simulink model "crane_sm"  (R2026a)
settings: Solver=ode23t  StopTime=8
undefined symbols (not defined in the file): ctrl_centerDamping, ctrl_centerGain, ctrl_clearanceMargin, ctrl_forceMax, ctrl_K, ctrl_lqrScale, ctrl_pendulumLength, ctrl_postClearDamping, ctrl_postClearGain, ctrl_pumpControlAmplitude, ctrl_pumpControlDuration, ctrl_pumpControlPhase, ctrl_pumpFrequency, ctrl_targetX, ctrl_transferClearance, ctrl_transferDamping, ctrl_transferForce, ctrl_wallTop, ctrl_wallX, X, Y, Z
libraries: sm_lib x18, nesl_utility x10
settings Model: DataDictionary=craneDD.sldd  Creator=grouleau  LastModifiedBy=grouleau

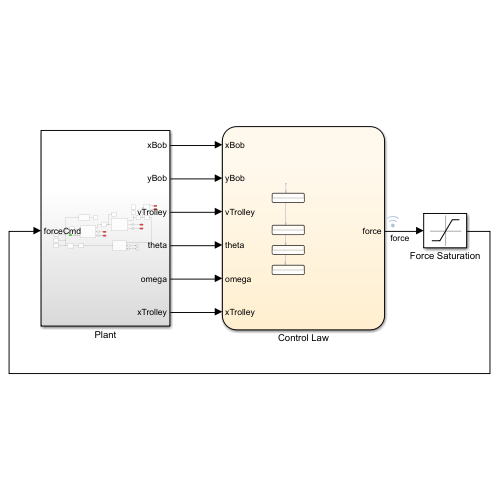
[thumbnail: Simulink's stored preview of the top-level diagram]
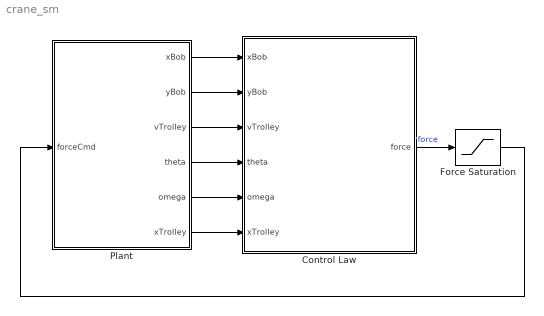
== system crane_sm ==
  Control Law : Stateflow chart  TreatAsAtomicUnit=on
  Force Saturation : Saturate  UpperLimit=60  LowerLimit=-60
  Plant : Subsystem
  wires:
  Plant/6(xTrolley) -> Control Law/6(xTrolley)
  Plant/5(omega) -> Control Law/5(omega)
  Control Law/1(force) -> Force Saturation/1  "force"
  Plant/4(theta) -> Control Law/4(theta)
  Plant/2(yBob) -> Control Law/2(yBob)
  Plant/3(vTrolley) -> Control Law/3(vTrolley)
  Plant/1(xBob) -> Control Law/1(xBob)
  Force Saturation/1 -> Plant/1(forceCmd)

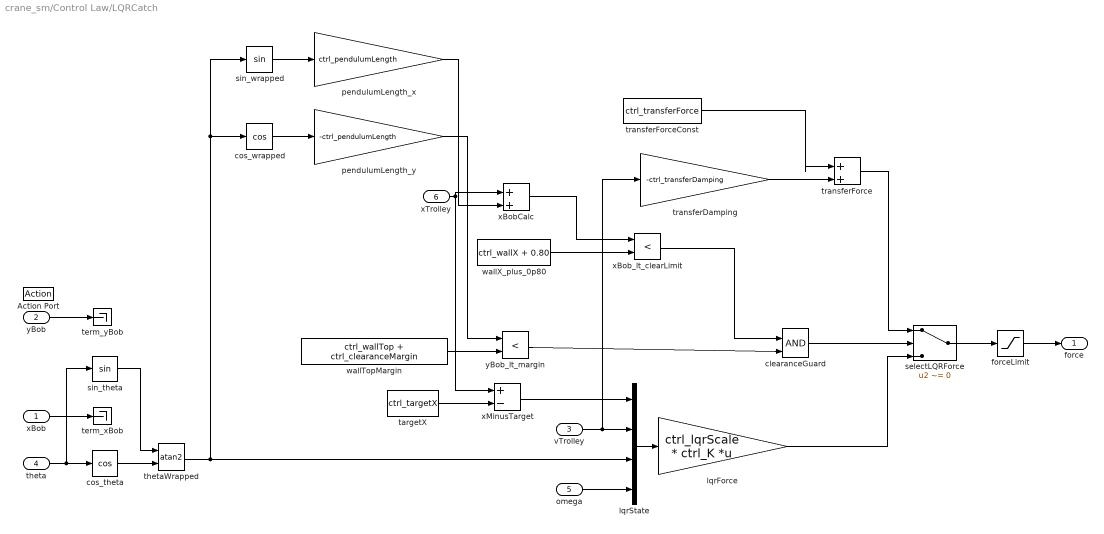
== system crane_sm/Control Law/LQRCatch ==
  xBob : Inport
  yBob : Inport  Port=2
  vTrolley : Inport  Port=3
  theta : Inport  Port=4
  omega : Inport  Port=5
  xTrolley : Inport  Port=6
  Action Port : ActionPort
      settings: CopyFcn=Stateflow.SLINSF.SimulinkMan.removeBlockPreDeleteFcn  PreDeleteFcn=Stateflow.SLINSF.SimulinkMan.unsafePredeleteFcn
  clearanceGuard : Logic  IconShape=distinctive  AllPortsSameDT=off  OutDataTypeStr=boolean
  cos_theta : Trigonometry  Operator=cos
  cos_wrapped : Trigonometry  Operator=cos
  forceLimit : Saturate  UpperLimit=ctrl_forceMax  LowerLimit=-ctrl_forceMax
  lqrForce : Gain  Gain=ctrl_lqrScale * ctrl_K  Multiplication=Matrix(K*u)
  lqrState : Mux
  pendulumLength_x : Gain  Gain=ctrl_pendulumLength
  pendulumLength_y : Gain  Gain=-ctrl_pendulumLength
  selectLQRForce : Switch  Criteria=u2 ~= 0  SaturateOnIntegerOverflow=off  InputSameDT=off
  sin_theta : Trigonometry
  sin_wrapped : Trigonometry
  targetX : Constant  Value=ctrl_targetX
  term_xBob : Terminator
  term_yBob : Terminator
  thetaWrapped : Trigonometry  Operator=atan2
  transferDamping : Gain  Gain=-ctrl_transferDamping
  transferForce : Sum  Inputs=|++
  transferForceConst : Constant  Value=ctrl_transferForce
  wallTopMargin : Constant  Value=ctrl_wallTop + ctrl_clearanceMargin
  wallX_plus_0p80 : Constant  Value=ctrl_wallX + 0.80
  xBobCalc : Sum  Inputs=|++
  xBob_lt_clearLimit : RelationalOperator  Operator=<  OutDataTypeStr=boolean  RndMeth=Simplest  InputSameDT=off
  xMinusTarget : Sum  Inputs=+-
  yBob_lt_margin : RelationalOperator  Operator=<  OutDataTypeStr=boolean  RndMeth=Simplest  InputSameDT=off
  force : Outport
  wires:
  yBob/1 -> term_yBob/1
  xBob/1 -> term_xBob/1
  omega/1 -> lqrState/4
  theta/1 -> sin_theta/1, cos_theta/1
  sin_theta/1 -> thetaWrapped/1
  thetaWrapped/1 -> sin_wrapped/1, cos_wrapped/1, lqrState/3
  sin_wrapped/1 -> pendulumLength_x/1
  cos_theta/1 -> thetaWrapped/2
  cos_wrapped/1 -> pendulumLength_y/1
  pendulumLength_x/1 -> xBobCalc/2
  wallX_plus_0p80/1 -> xBob_lt_clearLimit/2
  pendulumLength_y/1 -> yBob_lt_margin/1
  forceLimit/1 -> force/1
  xTrolley/1 -> xBobCalc/1, xMinusTarget/1
  xBob_lt_clearLimit/1 -> clearanceGuard/1
  wallTopMargin/1 -> yBob_lt_margin/2
  transferForce/1 -> selectLQRForce/1
  transferDamping/1 -> transferForce/2
  targetX/1 -> xMinusTarget/2
  xBobCalc/1 -> xBob_lt_clearLimit/1
  vTrolley/1 -> transferDamping/1, lqrState/2
  clearanceGuard/1 -> selectLQRForce/2
  transferForceConst/1 -> transferForce/1
  yBob_lt_margin/1 -> clearanceGuard/2
  lqrState/1 -> lqrForce/1
  xMinusTarget/1 -> lqrState/1
  lqrForce/1 -> selectLQRForce/3
  selectLQRForce/1 -> forceLimit/1

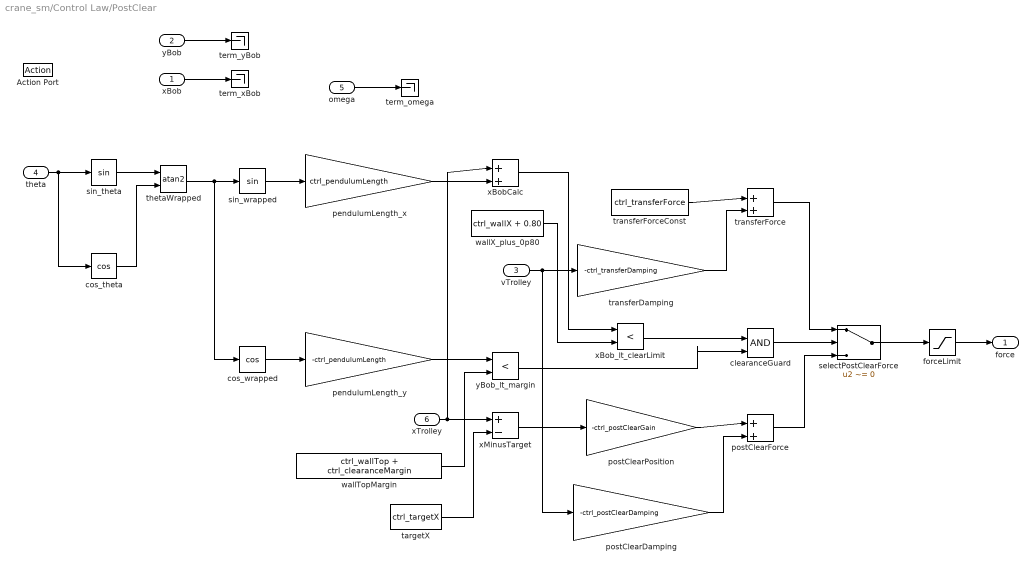
== system crane_sm/Control Law/PostClear ==
  xBob : Inport
  yBob : Inport  Port=2
  vTrolley : Inport  Port=3
  theta : Inport  Port=4
  omega : Inport  Port=5
  xTrolley : Inport  Port=6
  Action Port : ActionPort
      settings: CopyFcn=Stateflow.SLINSF.SimulinkMan.removeBlockPreDeleteFcn  PreDeleteFcn=Stateflow.SLINSF.SimulinkMan.unsafePredeleteFcn
  clearanceGuard : Logic  IconShape=distinctive  AllPortsSameDT=off  OutDataTypeStr=boolean
  cos_theta : Trigonometry  Operator=cos
  cos_wrapped : Trigonometry  Operator=cos
  forceLimit : Saturate  UpperLimit=ctrl_forceMax  LowerLimit=-ctrl_forceMax
  pendulumLength_x : Gain  Gain=ctrl_pendulumLength
  pendulumLength_y : Gain  Gain=-ctrl_pendulumLength
  postClearDamping : Gain  Gain=-ctrl_postClearDamping
  postClearForce : Sum  Inputs=|++
  postClearPosition : Gain  Gain=-ctrl_postClearGain
  selectPostClearForce : Switch  Criteria=u2 ~= 0  SaturateOnIntegerOverflow=off  InputSameDT=off
  sin_theta : Trigonometry
  sin_wrapped : Trigonometry
  targetX : Constant  Value=ctrl_targetX
  term_omega : Terminator
  term_xBob : Terminator
  term_yBob : Terminator
  thetaWrapped : Trigonometry  Operator=atan2
  transferDamping : Gain  Gain=-ctrl_transferDamping
  transferForce : Sum  Inputs=|++
  transferForceConst : Constant  Value=ctrl_transferForce
  wallTopMargin : Constant  Value=ctrl_wallTop + ctrl_clearanceMargin
  wallX_plus_0p80 : Constant  Value=ctrl_wallX + 0.80
  xBobCalc : Sum  Inputs=|++
  xBob_lt_clearLimit : RelationalOperator  Operator=<  OutDataTypeStr=boolean  RndMeth=Simplest  InputSameDT=off
  xMinusTarget : Sum  Inputs=+-
  yBob_lt_margin : RelationalOperator  Operator=<  OutDataTypeStr=boolean  RndMeth=Simplest  InputSameDT=off
  force : Outport
  wires:
  yBob/1 -> term_yBob/1
  xBob/1 -> term_xBob/1
  thetaWrapped/1 -> cos_wrapped/1, sin_wrapped/1
  cos_theta/1 -> thetaWrapped/2
  theta/1 -> sin_theta/1, cos_theta/1
  omega/1 -> term_omega/1
  sin_theta/1 -> thetaWrapped/1
  pendulumLength_x/1 -> xBobCalc/2
  sin_wrapped/1 -> pendulumLength_x/1
  cos_wrapped/1 -> pendulumLength_y/1
  pendulumLength_y/1 -> yBob_lt_margin/1
  xTrolley/1 -> xBobCalc/1, xMinusTarget/1
  xBob_lt_clearLimit/1 -> clearanceGuard/1
  wallX_plus_0p80/1 -> xBob_lt_clearLimit/2
  wallTopMargin/1 -> yBob_lt_margin/2
  xMinusTarget/1 -> postClearPosition/1
  targetX/1 -> xMinusTarget/2
  xBobCalc/1 -> xBob_lt_clearLimit/1
  vTrolley/1 -> transferDamping/1, postClearDamping/1
  clearanceGuard/1 -> selectPostClearForce/2
  yBob_lt_margin/1 -> clearanceGuard/2
  transferForceConst/1 -> transferForce/1
  transferForce/1 -> selectPostClearForce/1
  transferDamping/1 -> transferForce/2
  postClearPosition/1 -> postClearForce/1
  postClearForce/1 -> selectPostClearForce/3
  postClearDamping/1 -> postClearForce/2
  selectPostClearForce/1 -> forceLimit/1
  forceLimit/1 -> force/1

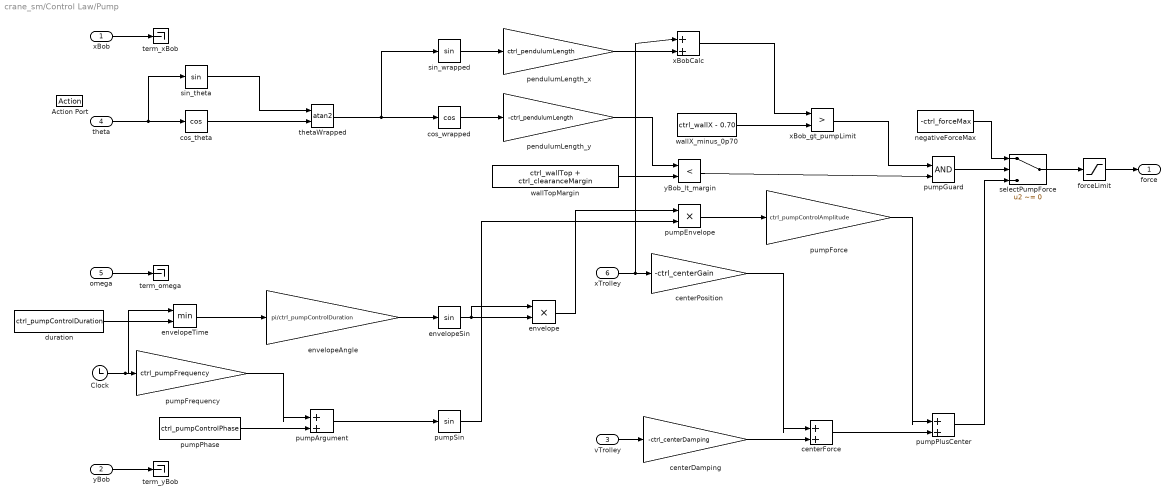
== system crane_sm/Control Law/Pump ==
  xBob : Inport
  yBob : Inport  Port=2
  vTrolley : Inport  Port=3
  theta : Inport  Port=4
  omega : Inport  Port=5
  xTrolley : Inport  Port=6
  Action Port : ActionPort
      settings: CopyFcn=Stateflow.SLINSF.SimulinkMan.removeBlockPreDeleteFcn  PreDeleteFcn=Stateflow.SLINSF.SimulinkMan.unsafePredeleteFcn
  Clock : Clock
  centerDamping : Gain  Gain=-ctrl_centerDamping
  centerForce : Sum  Inputs=|++
  centerPosition : Gain  Gain=-ctrl_centerGain
  cos_theta : Trigonometry  Operator=cos
  cos_wrapped : Trigonometry  Operator=cos
  duration : Constant  Value=ctrl_pumpControlDuration
  envelope : Product
  envelopeAngle : Gain  Gain=pi/ctrl_pumpControlDuration
  envelopeSin : Trigonometry
  envelopeTime : MinMax  Inputs=2
  forceLimit : Saturate  UpperLimit=ctrl_forceMax  LowerLimit=-ctrl_forceMax
  negativeForceMax : Constant  Value=-ctrl_forceMax
  pendulumLength_x : Gain  Gain=ctrl_pendulumLength
  pendulumLength_y : Gain  Gain=-ctrl_pendulumLength
  pumpArgument : Sum  Inputs=|++
  pumpEnvelope : Product
  pumpForce : Gain  Gain=ctrl_pumpControlAmplitude
  pumpFrequency : Gain  Gain=ctrl_pumpFrequency
  pumpGuard : Logic  IconShape=distinctive  AllPortsSameDT=off  OutDataTypeStr=boolean
  pumpPhase : Constant  Value=ctrl_pumpControlPhase
  pumpPlusCenter : Sum  Inputs=|++
  pumpSin : Trigonometry
  selectPumpForce : Switch  Criteria=u2 ~= 0  SaturateOnIntegerOverflow=off  InputSameDT=off
  sin_theta : Trigonometry
  sin_wrapped : Trigonometry
  term_omega : Terminator
  term_xBob : Terminator
  term_yBob : Terminator
  thetaWrapped : Trigonometry  Operator=atan2
  wallTopMargin : Constant  Value=ctrl_wallTop + ctrl_clearanceMargin
  wallX_minus_0p70 : Constant  Value=ctrl_wallX - 0.70
  xBobCalc : Sum  Inputs=|++
  xBob_gt_pumpLimit : RelationalOperator  Operator=>  OutDataTypeStr=boolean  RndMeth=Simplest  InputSameDT=off
  yBob_lt_margin : RelationalOperator  Operator=<  OutDataTypeStr=boolean  RndMeth=Simplest  InputSameDT=off
  force : Outport
  wires:
  duration/1 -> envelopeTime/2
  xBob/1 -> term_xBob/1
  yBob/1 -> term_yBob/1
  pendulumLength_x/1 -> xBobCalc/2
  theta/1 -> sin_theta/1, cos_theta/1
  omega/1 -> term_omega/1
  selectPumpForce/1 -> forceLimit/1
  Clock/1 -> envelopeTime/1, pumpFrequency/1
  sin_theta/1 -> thetaWrapped/1
  cos_theta/1 -> thetaWrapped/2
  envelopeTime/1 -> envelopeAngle/1
  pumpFrequency/1 -> pumpArgument/1
  pumpPhase/1 -> pumpArgument/2
  thetaWrapped/1 -> sin_wrapped/1, cos_wrapped/1
  envelopeSin/1 -> envelope/1, envelope/2
  envelopeAngle/1 -> envelopeSin/1
  pumpSin/1 -> pumpEnvelope/2
  pumpArgument/1 -> pumpSin/1
  sin_wrapped/1 -> pendulumLength_x/1
  cos_wrapped/1 -> pendulumLength_y/1
  xBobCalc/1 -> xBob_gt_pumpLimit/1
  pendulumLength_y/1 -> yBob_lt_margin/1
  wallTopMargin/1 -> yBob_lt_margin/2
  xTrolley/1 -> xBobCalc/1, centerPosition/1
  envelope/1 -> pumpEnvelope/1
  vTrolley/1 -> centerDamping/1
  pumpPlusCenter/1 -> selectPumpForce/3
  wallX_minus_0p70/1 -> xBob_gt_pumpLimit/2
  yBob_lt_margin/1 -> pumpGuard/2
  pumpEnvelope/1 -> pumpForce/1
  centerPosition/1 -> centerForce/1
  centerDamping/1 -> centerForce/2
  xBob_gt_pumpLimit/1 -> pumpGuard/1
  pumpForce/1 -> pumpPlusCenter/1
  centerForce/1 -> pumpPlusCenter/2
  pumpGuard/1 -> selectPumpForce/2
  negativeForceMax/1 -> selectPumpForce/1
  forceLimit/1 -> force/1

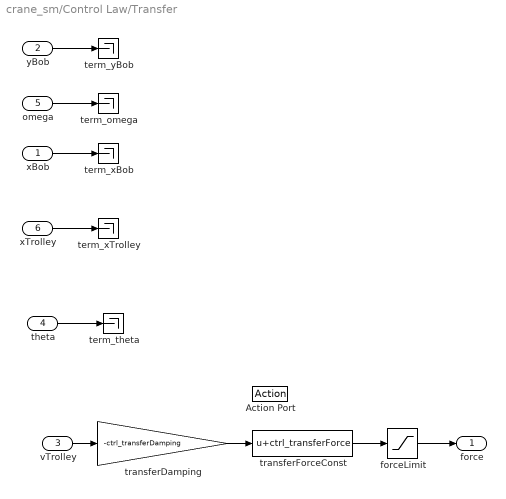
== system crane_sm/Control Law/Transfer ==
  xBob : Inport
  yBob : Inport  Port=2
  vTrolley : Inport  Port=3
  theta : Inport  Port=4
  omega : Inport  Port=5
  xTrolley : Inport  Port=6
  Action Port : ActionPort
      settings: CopyFcn=Stateflow.SLINSF.SimulinkMan.removeBlockPreDeleteFcn  PreDeleteFcn=Stateflow.SLINSF.SimulinkMan.unsafePredeleteFcn
  forceLimit : Saturate  UpperLimit=ctrl_forceMax  LowerLimit=-ctrl_forceMax
  term_omega : Terminator
  term_theta : Terminator
  term_xBob : Terminator
  term_xTrolley : Terminator
  term_yBob : Terminator
  transferDamping : Gain  Gain=-ctrl_transferDamping
  transferForceConst : Bias  Bias=ctrl_transferForce  SaturateOnIntegerOverflow=off
  force : Outport
  wires:
  yBob/1 -> term_yBob/1
  omega/1 -> term_omega/1
  theta/1 -> term_theta/1
  xBob/1 -> term_xBob/1
  xTrolley/1 -> term_xTrolley/1
  vTrolley/1 -> transferDamping/1
  transferForceConst/1 -> forceLimit/1
  transferDamping/1 -> transferForceConst/1
  forceLimit/1 -> force/1

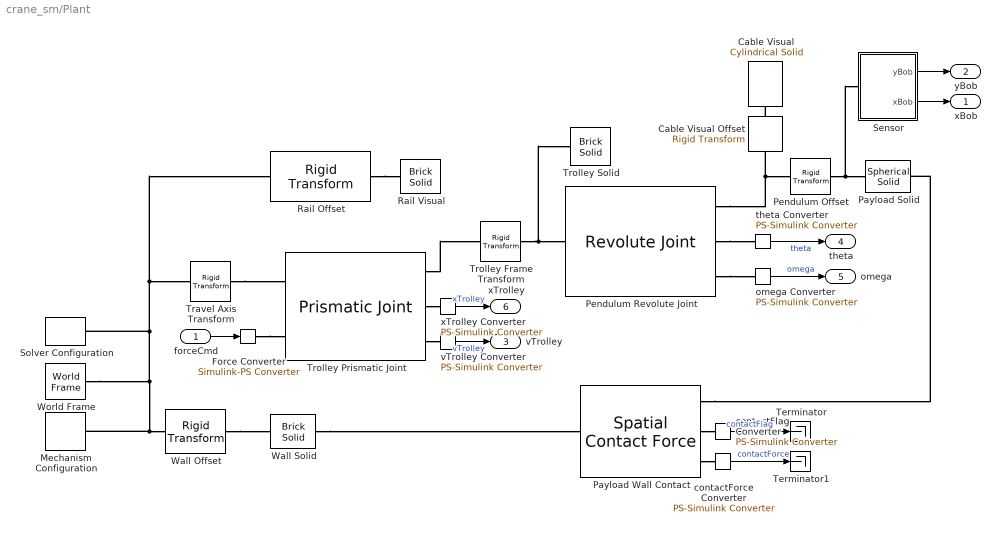
== system crane_sm/Plant ==
  forceCmd : Inport
  Cable Visual : sm_lib/Body Elements/Cylindrical Solid  CylinderRadius=0.015  CylinderRadiusUnits=m  CylinderLength=1.4  CylinderLengthUnits=m  ExportEntireGeometry=off  InertiaType=Custom  BasedOnType=Density  Density=1000  DensityUnits=kg/m^3  Mass=0  MassUnits=kg  CenterOfMass=[0 0 0]  CenterOfMassUnits=m  MomentsOfInertia=[0 0 0]  MomentsOfInertiaUnits=kg*m^2  ProductsOfInertia=[0 0 0]  ProductsOfInertiaUnits=kg*m^2  GraphicType=FromGeometry  MarkerShape=Sphere  MarkerSize=10  GraphicVisPropType=SimpleVisualProperties  GraphicDiffuseColor=[0.08 0.08 0.08]  GraphicOpacity=1  GraphicSpecularColor=[0.5 0.5 0.5 1.0]  GraphicAmbientColor=[0.15 0.15 0.15 1.0]  GraphicEmissiveColor=[0.0 0.0 0.0 1.0]  GraphicShininess=75  DoExposeReferenceFrame=on  SerializedFrames=<Frames/>
  Cable Visual Offset : sm_lib/Frames and Transforms/Rigid Transform  RotationMethod=StandardAxis  FollAlignAxisA=+X  BaseAlignAxisA=+Y  FollAlignAxisB=+Y  BaseAlignAxisB=+Z  RotationStandardAxis=+X  RotationAngle=90  RotationAngleUnits=deg  RotationArbitraryAxis=[0 0 1]  RotationSequenceAxes=FollowerAxes  RotationSequence=XYX  RotationSequenceAngles=[0 0 0]  RotationSequenceAnglesUnits=deg  RotationMatrix=[1 0 0;0 1 0;0 0 1]  Quaternion=[1 0 0 0]  TranslationMethod=Cartesian  TranslationCartesianOffset=[0 -0.7 0]  TranslationCartesianOffsetUnits=m  TranslationStandardAxis=+Z  TranslationStandardOffset=0  TranslationStandardOffsetUnits=m  TranslationROffset=0  TranslationROffsetUnits=m  TranslationThetaOffset=0  TranslationThetaOffsetUnits=deg  TranslationZOffset=0  TranslationZOffsetUnits=m
  Force Converter : nesl_utility/Simulink-PS Converter  PhysicalDomain=network_engine_domain  SubClassName=ps_input  LeftPortType=input  RightPortType=output  PseudoPeriodic=off  Frequencies=[]  NoiseDistribution=none  NoiseParameters=[]  Unit=N  AffineConversion=off  FilteringAndDerivatives=provide  SimscapeFilterOrder=1  InputFilterTimeConstant=0.001  UdotUserProvided=0
  Mechanism Configuration : sm_lib/Utilities/Mechanism Configuration  UniformGravity=Constant  GravityVector=[0 -9.81 0]  GravityVectorUnits=m/s^2  LinearizationDelta=0.001  JointModeTransitionNonlinearIterations=2
  Payload Solid : sm_lib/Body Elements/Spherical Solid  SphereRadius=0.12  SphereRadiusUnits=m  ExportEntireGeometry=on  InertiaType=Custom  BasedOnType=Density  Density=1000  DensityUnits=kg/m^3  Mass=1.5  MassUnits=kg  CenterOfMass=[0 0 0]  CenterOfMassUnits=m  MomentsOfInertia=[1 1 1]  MomentsOfInertiaUnits=kg*m^2  ProductsOfInertia=[0 0 0]  ProductsOfInertiaUnits=kg*m^2  GraphicType=FromGeometry  MarkerShape=Sphere  MarkerSize=10  GraphicVisPropType=SimpleVisualProperties  GraphicDiffuseColor=[0.85 0.33 0.10]  GraphicOpacity=1  GraphicSpecularColor=[0.5 0.5 0.5 1.0]  GraphicAmbientColor=[0.15 0.15 0.15 1.0]  GraphicEmissiveColor=[0.0 0.0 0.0 1.0]  GraphicShininess=75  DoExposeReferenceFrame=on  SerializedFrames=<Frames/>
  Payload Wall Contact : sm_lib/Forces and Torques/Spatial Contact Force  SenseSeparationDistance=off  NormalForceType=SmoothSpringDamper  NormalStiffness=1000  NormalStiffnessUnits=N/m  NormalDamping=100  NormalDampingUnits=N/(m/s)  NormalTransitionRegionWidth=0.001  NormalTransitionRegionWidthUnits=m  FrictionType=SmoothStickSlip  CoefficientOfStaticFriction=0.5  CoefficientOfDynamicFriction=0.3  FrictionalCriticalVelocity=1e-3  FrictionalCriticalVelocityUnits=m/s  SenseContactSignal=on  SensePenetrationDepth=off  SenseNormalVelocity=off  SenseTangentialVelocity=off  SensingForceTorqueDirection=BaseOnFollower  SensingForceTorqueResolutionFrame=ContactFrame  SenseNormalForce=off  SenseNormalForceMagnitude=on  SenseNormalTorque=off  SenseFrictionalForce=off  SenseFrictionalForceMagnitude=off  SenseFrictionalTorque=off  SenseTotalForce=off  SenseTotalTorque=off  SenseContactBaseRotation=off  SenseContactBaseTranslation=off  SenseContactFollowerRotation=off  SenseContactFollowerTranslation=off  ZeroCrossDetectContactStartAndEnd=off
  Pendulum Offset : sm_lib/Frames and Transforms/Rigid Transform  RotationMethod=None  FollAlignAxisA=+X  BaseAlignAxisA=+Y  FollAlignAxisB=+Y  BaseAlignAxisB=+Z  RotationStandardAxis=+Z  RotationAngle=0  RotationAngleUnits=deg  RotationArbitraryAxis=[0 0 1]  RotationSequenceAxes=FollowerAxes  RotationSequence=XYX  RotationSequenceAngles=[0 0 0]  RotationSequenceAnglesUnits=deg  RotationMatrix=[1 0 0;0 1 0;0 0 1]  Quaternion=[1 0 0 0]  TranslationMethod=Cartesian  TranslationCartesianOffset=[0 -1.4 0]  TranslationCartesianOffsetUnits=m  TranslationStandardAxis=+Z  TranslationStandardOffset=0  TranslationStandardOffsetUnits=m  TranslationROffset=0  TranslationROffsetUnits=m  TranslationThetaOffset=0  TranslationThetaOffsetUnits=deg  TranslationZOffset=0  TranslationZOffsetUnits=m
  Pendulum Revolute Joint : sm_lib/Joints/Revolute Joint  JointMode=Normal  CompositeWrenchDir=FollowerOnBase  CompositeWrenchFrame=BaseFrame  SenseConstraintForce=off  SenseConstraintTorque=off  SenseTotalForce=off  SenseTotalTorque=off  PositionTargetSpecify=on  PositionTargetPriority=High  PositionTargetValue=0  PositionTargetValueUnits=deg  VelocityTargetSpecify=off  VelocityTargetPriority=High  VelocityTargetValue=0  VelocityTargetValueUnits=deg/s  EquilibriumPosition=0  EquilibriumPositionUnits=deg  SpringStiffness=0  SpringStiffnessUnits=N*m/deg  DampingCoefficient=0  DampingCoefficientUnits=N*m/(deg/s)  LowerLimitSpecify=off  LowerLimitBound=-90  LowerLimitBoundUnits=deg  LowerLimitStiffness=1e4  LowerLimitStiffnessUnits=N*m/deg  LowerLimitDamping=10  LowerLimitDampingUnits=N*m/(deg/s)  LowerLimitTransitionRegionWidth=0.1  LowerLimitTransitionRegionWidthUnits=deg  UpperLimitSpecify=off  UpperLimitBound=90  UpperLimitBoundUnits=deg  UpperLimitStiffness=1e4  UpperLimitStiffnessUnits=N*m/deg  UpperLimitDamping=10  UpperLimitDampingUnits=N*m/(deg/s)  UpperLimitTransitionRegionWidth=0.1  UpperLimitTransitionRegionWidthUnits=deg  TorqueActuationMode=NoTorque  MotionActuationMode=ComputedMotion  SensePosition=on  SenseVelocity=on  SenseAcceleration=off  SenseTorqueForce=off  SenseLowerLimitTorqueForce=off  SenseUpperLimitTorqueForce=off
  Rail Offset : sm_lib/Frames and Transforms/Rigid Transform  RotationMethod=None  FollAlignAxisA=+X  BaseAlignAxisA=+Y  FollAlignAxisB=+Y  BaseAlignAxisB=+Z  RotationStandardAxis=+Z  RotationAngle=0  RotationAngleUnits=deg  RotationArbitraryAxis=[0 0 1]  RotationSequenceAxes=FollowerAxes  RotationSequence=XYX  RotationSequenceAngles=[0 0 0]  RotationSequenceAnglesUnits=deg  RotationMatrix=[1 0 0;0 1 0;0 0 1]  Quaternion=[1 0 0 0]  TranslationMethod=Cartesian  TranslationCartesianOffset=[0 0 0]  TranslationCartesianOffsetUnits=m  TranslationStandardAxis=+Z  TranslationStandardOffset=0  TranslationStandardOffsetUnits=m  TranslationROffset=0  TranslationROffsetUnits=m  TranslationThetaOffset=0  TranslationThetaOffsetUnits=deg  TranslationZOffset=0  TranslationZOffsetUnits=m
  Rail Visual : sm_lib/Body Elements/Brick Solid  BrickDimensions=[10 0.08 0.08]  BrickDimensionsUnits=m  ExportEntireGeometry=off  InertiaType=Custom  BasedOnType=Density  Density=1000  DensityUnits=kg/m^3  Mass=1  MassUnits=kg  CenterOfMass=[0 0 0]  CenterOfMassUnits=m  MomentsOfInertia=[1 1 1]  MomentsOfInertiaUnits=kg*m^2  ProductsOfInertia=[0 0 0]  ProductsOfInertiaUnits=kg*m^2  GraphicType=FromGeometry  MarkerShape=Sphere  MarkerSize=10  GraphicVisPropType=SimpleVisualProperties  GraphicDiffuseColor=[0.35 0.35 0.35]  GraphicOpacity=1  GraphicSpecularColor=[0.5 0.5 0.5 1.0]  GraphicAmbientColor=[0.15 0.15 0.15 1.0]  GraphicEmissiveColor=[0.0 0.0 0.0 1.0]  GraphicShininess=75  DoExposeReferenceFrame=on  SerializedFrames=<Frames/>
  Sensor : Subsystem
  Solver Configuration : nesl_utility/Solver Configuration  PhysicalDomain=network_engine_domain  SubClassName=solver  LeftPortType=input  RightPortType=generic  Tones=[]  Harmonics=[]  SimulateNoise=off  Profile=off  UseLocalSampling=off  EnableSwitchedLinearOptims=on  FrequencyDomain=off  UseCCode=off  RelTol=0.001  AbsTol=0.001  MinStep=1e-09  ToWorkspace=off  RevertToSquareIcSolve=off  NumHomotopyIterations=100  PhasorMode=off  PhasorModeNumHarmonics=1  ConsistencySolver=NEWTON_XTOL_AFTER_FTOL  CanonicalOrdering=CANONICAL  OptimizeIntermediates=OPTIMIZED  IndexReductionMethod=DerivativeReplacement  DoDC=off  ResidualTolerance=1e-09  ConsistencyTolSource=GLOBAL  ConsistencyAbsTol=0.001  ConsistencyRelTol=0.001  ConsistencyTolFactor=0.001  UseLocalSolver=off  LocalSolverChoice=NE_BACKWARD_EULER_ADVANCER  ResolveIndetEquations=on  FunctionEvalNumThread=1  LocalSolverSampleTime=0.001  DoFixedCost=off  MaxNonlinIter=3  MaxModeIter=2  ComputeImpulses=off  ImpulseIterations=2  LinearAlgebra=auto  LinearAlgebraNumThread=0  EquationFormulation=NE_TIME_EF  DelaysMemoryBudget=1024  AutomaticFiltering=on  FilteringTimeConstant=0.001  PartitionStorageMethod=AS_NEEDED  PartitionMemoryBudget=1024  PartitionMethod=ROBUST  MultibodyUseLocalSolver=off  MultibodyLocalSolverChoice=ODE1  MultibodyLocalSolverSampleTime=0.001
  Terminator : Terminator
  Terminator1 : Terminator
  Travel Axis Transform : sm_lib/Frames and Transforms/Rigid Transform  RotationMethod=StandardAxis  FollAlignAxisA=+X  BaseAlignAxisA=+Y  FollAlignAxisB=+Y  BaseAlignAxisB=+Z  RotationStandardAxis=+Y  RotationAngle=90  RotationAngleUnits=deg  RotationArbitraryAxis=[0 0 1]  RotationSequenceAxes=FollowerAxes  RotationSequence=XYX  RotationSequenceAngles=[0 0 0]  RotationSequenceAnglesUnits=deg  RotationMatrix=[1 0 0;0 1 0;0 0 1]  Quaternion=[1 0 0 0]  TranslationMethod=None  TranslationCartesianOffset=[0 0 0]  TranslationCartesianOffsetUnits=m  TranslationStandardAxis=+Z  TranslationStandardOffset=0  TranslationStandardOffsetUnits=m  TranslationROffset=0  TranslationROffsetUnits=m  TranslationThetaOffset=0  TranslationThetaOffsetUnits=deg  TranslationZOffset=0  TranslationZOffsetUnits=m
  Trolley Frame Transform : sm_lib/Frames and Transforms/Rigid Transform  RotationMethod=StandardAxis  FollAlignAxisA=+X  BaseAlignAxisA=+Y  FollAlignAxisB=+Y  BaseAlignAxisB=+Z  RotationStandardAxis=+Y  RotationAngle=-90  RotationAngleUnits=deg  RotationArbitraryAxis=[0 0 1]  RotationSequenceAxes=FollowerAxes  RotationSequence=XYX  RotationSequenceAngles=[0 0 0]  RotationSequenceAnglesUnits=deg  RotationMatrix=[1 0 0;0 1 0;0 0 1]  Quaternion=[1 0 0 0]  TranslationMethod=None  TranslationCartesianOffset=[0 0 0]  TranslationCartesianOffsetUnits=m  TranslationStandardAxis=+Z  TranslationStandardOffset=0  TranslationStandardOffsetUnits=m  TranslationROffset=0  TranslationROffsetUnits=m  TranslationThetaOffset=0  TranslationThetaOffsetUnits=deg  TranslationZOffset=0  TranslationZOffsetUnits=m
  Trolley Prismatic Joint : sm_lib/Joints/Prismatic Joint  JointMode=Normal  CompositeWrenchDir=FollowerOnBase  CompositeWrenchFrame=BaseFrame  SenseConstraintForce=off  SenseConstraintTorque=off  SenseTotalForce=off  SenseTotalTorque=off  PositionTargetSpecify=off  PositionTargetPriority=High  PositionTargetValue=0  PositionTargetValueUnits=m  VelocityTargetSpecify=off  VelocityTargetPriority=High  VelocityTargetValue=0  VelocityTargetValueUnits=m/s  EquilibriumPosition=0  EquilibriumPositionUnits=m  SpringStiffness=0  SpringStiffnessUnits=N/m  DampingCoefficient=0  DampingCoefficientUnits=N/(m/s)  LowerLimitSpecify=off  LowerLimitBound=-1  LowerLimitBoundUnits=m  LowerLimitStiffness=1e6  LowerLimitStiffnessUnits=N/m  LowerLimitDamping=1e3  LowerLimitDampingUnits=N/(m/s)  LowerLimitTransitionRegionWidth=1e-4  LowerLimitTransitionRegionWidthUnits=m  UpperLimitSpecify=off  UpperLimitBound=1  UpperLimitBoundUnits=m  UpperLimitStiffness=1e6  UpperLimitStiffnessUnits=N/m  UpperLimitDamping=1e3  UpperLimitDampingUnits=N/(m/s)  UpperLimitTransitionRegionWidth=1e-4  UpperLimitTransitionRegionWidthUnits=m  TorqueActuationMode=InputTorque  MotionActuationMode=ComputedMotion  SensePosition=on  SenseVelocity=on  SenseAcceleration=off  SenseTorqueForce=off  SenseLowerLimitTorqueForce=off  SenseUpperLimitTorqueForce=off
  Trolley Solid : sm_lib/Body Elements/Brick Solid  BrickDimensions=[0.35 0.2 0.25]  BrickDimensionsUnits=m  ExportEntireGeometry=off  InertiaType=Custom  BasedOnType=Density  Density=1000  DensityUnits=kg/m^3  Mass=8  MassUnits=kg  CenterOfMass=[0 0 0]  CenterOfMassUnits=m  MomentsOfInertia=[1 1 1]  MomentsOfInertiaUnits=kg*m^2  ProductsOfInertia=[0 0 0]  ProductsOfInertiaUnits=kg*m^2  GraphicType=FromGeometry  MarkerShape=Sphere  MarkerSize=10  GraphicVisPropType=SimpleVisualProperties  GraphicDiffuseColor=[0.0 0.45 0.74]  GraphicOpacity=1  GraphicSpecularColor=[0.5 0.5 0.5 1.0]  GraphicAmbientColor=[0.15 0.15 0.15 1.0]  GraphicEmissiveColor=[0.0 0.0 0.0 1.0]  GraphicShininess=75  DoExposeReferenceFrame=on  SerializedFrames=<Frames/>
  Wall Offset : sm_lib/Frames and Transforms/Rigid Transform  RotationMethod=None  FollAlignAxisA=+X  BaseAlignAxisA=+Y  FollAlignAxisB=+Y  BaseAlignAxisB=+Z  RotationStandardAxis=+Z  RotationAngle=0  RotationAngleUnits=deg  RotationArbitraryAxis=[0 0 1]  RotationSequenceAxes=FollowerAxes  RotationSequence=XYX  RotationSequenceAngles=[0 0 0]  RotationSequenceAnglesUnits=deg  RotationMatrix=[1 0 0;0 1 0;0 0 1]  Quaternion=[1 0 0 0]  TranslationMethod=Cartesian  TranslationCartesianOffset=[1.45 -1.4 0]  TranslationCartesianOffsetUnits=m  TranslationStandardAxis=+Z  TranslationStandardOffset=0  TranslationStandardOffsetUnits=m  TranslationROffset=0  TranslationROffsetUnits=m  TranslationThetaOffset=0  TranslationThetaOffsetUnits=deg  TranslationZOffset=0  TranslationZOffsetUnits=m
  Wall Solid : sm_lib/Body Elements/Brick Solid  BrickDimensions=[0.1 1 2]  BrickDimensionsUnits=m  ExportEntireGeometry=on  InertiaType=Custom  BasedOnType=Density  Density=1000  DensityUnits=kg/m^3  Mass=50  MassUnits=kg  CenterOfMass=[0 0 0]  CenterOfMassUnits=m  MomentsOfInertia=[1 1 1]  MomentsOfInertiaUnits=kg*m^2  ProductsOfInertia=[0 0 0]  ProductsOfInertiaUnits=kg*m^2  GraphicType=FromGeometry  MarkerShape=Sphere  MarkerSize=10  GraphicVisPropType=SimpleVisualProperties  GraphicDiffuseColor=[0 1 0]  GraphicOpacity=1  GraphicSpecularColor=[0.5 0.5 0.5 1.0]  GraphicAmbientColor=[0.15 0.15 0.15 1.0]  GraphicEmissiveColor=[0.0 0.0 0.0 1.0]  GraphicShininess=75  DoExposeReferenceFrame=on  SerializedFrames=<Frames/>
  World Frame : sm_lib/Frames and Transforms/World Frame
  contactFlag Converter : nesl_utility/PS-Simulink Converter  PhysicalDomain=network_engine_domain  SubClassName=ps_output  LeftPortType=input  RightPortType=output  PseudoPeriodic=off  Frequencies=[]  VectorFormat=inherit  Unit=1  AffineConversion=off
  contactForce Converter : nesl_utility/PS-Simulink Converter  PhysicalDomain=network_engine_domain  SubClassName=ps_output  LeftPortType=input  RightPortType=output  PseudoPeriodic=off  Frequencies=[]  VectorFormat=inherit  Unit=N  AffineConversion=off
  omega Converter : nesl_utility/PS-Simulink Converter  PhysicalDomain=network_engine_domain  SubClassName=ps_output  LeftPortType=input  RightPortType=output  PseudoPeriodic=off  Frequencies=[]  VectorFormat=inherit  Unit=rad/s  AffineConversion=off
  theta Converter : nesl_utility/PS-Simulink Converter  PhysicalDomain=network_engine_domain  SubClassName=ps_output  LeftPortType=input  RightPortType=output  PseudoPeriodic=off  Frequencies=[]  VectorFormat=inherit  Unit=rad  AffineConversion=off
  vTrolley Converter : nesl_utility/PS-Simulink Converter  PhysicalDomain=network_engine_domain  SubClassName=ps_output  LeftPortType=input  RightPortType=output  PseudoPeriodic=off  Frequencies=[]  VectorFormat=inherit  Unit=m/s  AffineConversion=off
  xTrolley Converter : nesl_utility/PS-Simulink Converter  PhysicalDomain=network_engine_domain  SubClassName=ps_output  LeftPortType=input  RightPortType=output  PseudoPeriodic=off  Frequencies=[]  VectorFormat=inherit  Unit=m  AffineConversion=off
  xBob : Outport
  yBob : Outport  Port=2
  vTrolley : Outport  Port=3
  theta : Outport  Port=4
  omega : Outport  Port=5
  xTrolley : Outport  Port=6
  wires:
  forceCmd/1 -> Force Converter/1
  xTrolley Converter/1 -> xTrolley/1  "xTrolley"
  vTrolley Converter/1 -> vTrolley/1  "vTrolley"
  theta Converter/1 -> theta/1  "theta"
  omega Converter/1 -> omega/1  "omega"
  contactFlag Converter/1 -> Terminator/1  "contactFlag"
  contactForce Converter/1 -> Terminator1/1  "contactForce"
  Sensor/1(yBob) -> yBob/1
  Sensor/2(xBob) -> xBob/1
  connections:
  Wall Offset/RConn1 -- Wall Solid/RConn1
  World Frame/RConn1 -- Wall Offset/LConn1 -- Mechanism Configuration/RConn1 -- Rail Offset/LConn1 -- Travel Axis Transform/LConn1 -- Solver Configuration/RConn1
  Pendulum Offset/RConn1 -- Sensor/LConn1 -- Payload Solid/RConn1
  Pendulum Revolute Joint/RConn2 -- theta Converter/LConn1
  Rail Offset/RConn1 -- Rail Visual/RConn1
  Force Converter/RConn1 -- Trolley Prismatic Joint/LConn2
  Travel Axis Transform/RConn1 -- Trolley Prismatic Joint/LConn1
  Trolley Prismatic Joint/RConn2 -- xTrolley Converter/LConn1
  Trolley Frame Transform/RConn1 -- Trolley Solid/RConn1 -- Pendulum Revolute Joint/LConn1
  Trolley Prismatic Joint/RConn1 -- Trolley Frame Transform/LConn1
  Trolley Prismatic Joint/RConn3 -- vTrolley Converter/LConn1
  Pendulum Revolute Joint/RConn1 -- Pendulum Offset/LConn1 -- Cable Visual Offset/LConn1
  Pendulum Revolute Joint/RConn3 -- omega Converter/LConn1
  Cable Visual Offset/RConn1 -- Cable Visual/RConn1
  Payload Wall Contact/RConn3 -- contactForce Converter/LConn1
  Payload Wall Contact/RConn2 -- contactFlag Converter/LConn1
  Wall Solid/LConn1 -- Payload Wall Contact/LConn1
  Payload Wall Contact/RConn1 -- Payload Solid/LConn1

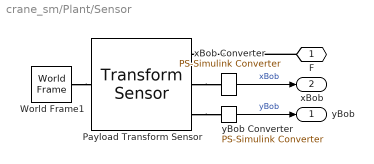
== system crane_sm/Plant/Sensor ==
  Payload Transform Sensor : sm_lib/Frames and Transforms/Transform Sensor  MeasurementFrame=World  RotationSequence=XYX  SenseAngle=off  SenseAxis=off  SenseQ=off  SenseR=off  SenseRotationSequence=off  SenseOmegaX=off  SenseOmegaY=off  SenseOmegaZ=off  SenseOmega=off  SenseQDot=off  SenseRDot=off  SenseRotationSequenceDot=off  SenseAlphaX=off  SenseAlphaY=off  SenseAlphaZ=off  SenseAlpha=off  SenseQDDot=off  SenseRDDot=off  SenseX=on  SenseY=on  SenseZ=off  SenseXYZ=off  SenseRad=off  SenseAzim=off  SenseDist=off  SenseInc=off  SenseXDot=off  SenseYDot=off  SenseZDot=off  SenseXYZDot=off  SenseRadDot=off  SenseAzimDot=off  SenseDistDot=off  SenseIncDot=off  SenseXDDot=off  SenseYDDot=off  SenseZDDot=off  SenseXYZDDot=off  SenseRadDDot=off  SenseAzimDDot=off  SenseDistDDot=off  SenseIncDDot=off
  World Frame1 : sm_lib/Frames and Transforms/World Frame
  xBob Converter : nesl_utility/PS-Simulink Converter  PhysicalDomain=network_engine_domain  SubClassName=ps_output  LeftPortType=input  RightPortType=output  PseudoPeriodic=off  Frequencies=[]  VectorFormat=inherit  Unit=m  AffineConversion=off
  yBob Converter : nesl_utility/PS-Simulink Converter  PhysicalDomain=network_engine_domain  SubClassName=ps_output  LeftPortType=input  RightPortType=output  PseudoPeriodic=off  Frequencies=[]  VectorFormat=inherit  Unit=m  AffineConversion=off
  F : PMIOPort  Side=Left
  yBob : Outport
  xBob : Outport  Port=2
  wires:
  xBob Converter/1 -> xBob/1  "xBob"
  yBob Converter/1 -> yBob/1  "yBob"
  connections:
  Payload Transform Sensor/RConn3 -- yBob Converter/LConn1
  World Frame1/RConn1 -- Payload Transform Sensor/LConn1
  F/RConn1 -- Payload Transform Sensor/RConn1
  Payload Transform Sensor/RConn2 -- xBob Converter/LConn1

== stateflow chart crane_sm/Control Law ==
  state Pump
  state Transfer
  state PostClear
  state LQRCatch
  (default) -> Pump
  Pump -> Transfer : [t > 1 && yBob > ctrl_wallTop + ctrl_transferClearance &&...
      |  xBob < ctrl_wallX &&...
      |  (vTrolley + ctrl_pendulumLength*cos(atan2(sin(theta),cos(theta)))*omega) > 0]
  Transfer -> PostClear : [xBob > ctrl_wallX + 0.35]
  PostClear -> LQRCatch : [abs(atan2(sin(theta),cos(theta))) < 0.9 && abs(omega) < 2.5]
  data: sf_internal_action_state_placeholder_data local double size=1 =0; sf_internal_action_state_placeholder_data local double size=1 =0; sf_internal_action_state_placeholder_data local double size=1 =0; sf_internal_action_state_placeholder_data local double size=1 =0; xBob input; yBob input; vTrolley input; theta input; omega input; force output; ctrl_wallX parameter; ctrl_wallTop parameter; ctrl_transferClearance parameter; ctrl_pendulumLength parameter; xTrolley input
